simulink library "Lib_Solve_SSNRSolverBroydUpdate_TMATS"  (R2021b)
settings: Solver=ode45  StartTime=0.0  StopTime=10.0  RelTol=1e-3  EnableMultiTasking=on
libraries: Lib_NM_JacobianCalc_TMATS x1
Description:
  | Thomas Modules
settings Model: Creator=jwchapm2  LastModifiedBy=jwchapm2
settings SolverCC: AlgebraicLoopSolver=TrustRegion
settings DataIOCC: LimitDataPoints=on  SaveFormat=Array  ReturnWorkspaceOutputs=off
settings OptimizationCC: ExpressionDepthLimit=2147483647  LifeSpan=inf
settings DebuggingCC: UnderspecifiedInitializationDetection=Classic  MergeDetectMultiDrivingBlocksExec=none  SolverPrmCheckMsg=warning  StateNameClashWarn=warning  SFUnexpectedBacktrackingDiag=warning  SFNoUnconditionalDefaultTransitionDiag=warning  SFExecutionAtInitializationDiag=none  ArithmeticOperatorsInVariantConditions=warning
settings HardwareCC: ProdBitPerPointer=32  ProdBitPerSizeT=32  ProdBitPerPtrDiffT=32  ProdLargestAtomicFloat=None  ProdIntDivRoundTo=Undefined  ProdEndianess=Unspecified  ProdWordSize=32  ProdHWDeviceType=32-bit Generic
settings ModelReferenceCC: PropagateSignalLabelsOutOfModel=off
settings SFSimCC: SimUseLocalCustomCode=off  CustomCodeUndefinedFunction=UseInterfaceOnly
settings RTWCC: RTWUseLocalCustomCode=off
settings CodeAppCC: StateflowObjectComments=on
settings GRTTargetCC: TargetLangStandard=C89/C90 (ANSI)
settings ConfigComp: CovMetricSettings=dw  CovSaveCumulativeToWorkspaceVar=on  CovSaveSingleToWorkspaceVar=on  CovExternalEMLEnable=off

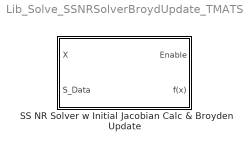
== system Lib_Solve_SSNRSolverBroydUpdate_TMATS ==
  SS NR Solver w Initial Jacobian Calc & Broyden Update : Subsystem  mask(T-MATS: SS NR Solver w Initial Jacobian Calc and Broyden Update Library Block){SJac_Per_M=[0.01 0.01 0.01;-0.01 -0.01,-0.01], SNR_IC_M=[1; 2; 3], SNR_DX_M=100, SNR_Mx_M=1000000, SNR_Mn_M=-1000000, Cond_Limits_M=0.0001}
      mask prompts: SJac_Per_M "SJac_Per_M - Jacobian Perturbation size (frac)(nxm)"; SNR_IC_M "SNR_IC_M - Newton Raphson Initial Conditions (mx1)"; SNR_DX_M "SNR_DX_M - Newton Raphson step size dampener. Percentage of calculated dx to use for each step (%) (1x1)"; SNR_Mx_M "SNR_Mx_M - Newton Raphson max limit (1x1 or mx1)"; SNR_Mn_M "SNR_Mn_M - Newton Raphson min limit (1x1 or mx1)"; Cond_Limits_M "Cond_Limits_M - Iteration Conditions Limits (mx1 or 1x1)"
      mask help:
      | The Steady State Newton Raphson Solver with Initial Jacobian Calculator and Broyden Update Method block will
      | supply the inputs to iteratively drive the outputs of a system to zero.
      |
      | This will be performed in three steps.
      | 1) Jabobian calculator sends Perturbations to the plant then calculates the initial plant
      | Jacboian based on the system response.
      | 2) The Newton Raphson Solver will use the inverse of the Jacobian to iteratively step the
      | system toward solution.
      | 3) The inverse of the Jacobian will be updated at each iteration via the Sherman-Morrison (Good) Broyden Update Method.
      | 3) Once the solution has satisfied the conditions the Newton Raphson Solver is shut off.
      |
      | Simulation run time length should be selected as to give the Newton Raphson Solver adequate time to develop a solution.
      mask init:
      | if isequal(size(SNR_Mx_M),size(SNR_IC_M))
      | elseif isequal(size(SNR_Mx_M),[1 1])
      | else
      |     disp('NR_Mx_Lim_M must be the same size as NR_IC_M or a constant')
      | end
      | 
      | if isequal(size(SNR_Mn_M),size(SNR_IC_M))
      | elseif isequal(size(SNR_Mn_M),[1 1])
      | else
      |     disp('NR_Mn_Lim_M must be the same size as NR_IC_M or a constant')
      | end
      mask Help: web(which('Solver_TMATS_SSNRwBU.html'),'-helpbrowser')

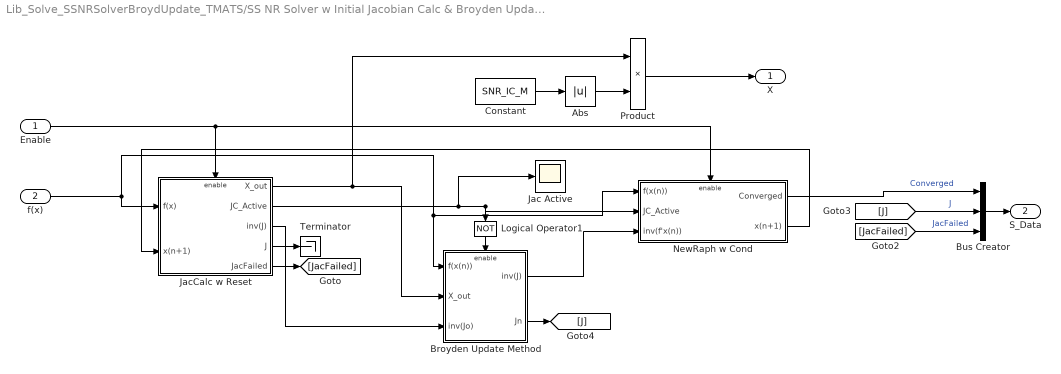
== system Lib_Solve_SSNRSolverBroydUpdate_TMATS/SS NR Solver w Initial Jacobian Calc & Broyden Update ==
  Enable : Inport  PortDimensions=1
  f(x) : Inport  Port=2  PortDimensions=length(SNR_IC_M)
  Abs : Abs
  Broyden Update Method : Subsystem
  Bus Creator : BusCreator  Inputs=3
  Constant : Constant  Value=SNR_IC_M
  Jac Active : Scope
  JacCalc w Reset : Subsystem  TreatAsAtomicUnit=on
  Logical Operator1 : Logic  Operator=NOT  AllPortsSameDT=off  OutDataTypeStr=boolean
  NewRaph w Cond : Subsystem  TreatAsAtomicUnit=on
  Product : Product  RndMeth=Zero
  Terminator : Terminator
  X : Outport  PortDimensions=length(SNR_IC_M)
  S_Data : Outport  Port=2  PortDimensions={1,[length(SNR_IC_M),length(SNR_IC_M)]}
  wires:
  Broyden Update Method/1("inv(J) ") -> NewRaph w Cond/3(inv(f'x(n)))
  Abs/1 -> Product/2
  Constant/1 -> Abs/1
  Product/1 -> X/1
  JacCalc w Reset/1(X_out) -> Broyden Update Method/2(X_out), Product/1
  Logical Operator1/1 -> Broyden Update Method/Enable
  Broyden Update Method/2(Jn) -> [J]
  JacCalc w Reset/2(JC_Active) -> NewRaph w Cond/2(JC_Active), Logical Operator1/1, Jac Active/1
  JacCalc w Reset/3(inv(J)) -> Broyden Update Method/3(inv(Jo))
  JacCalc w Reset/4(J) -> Terminator/1
  f(x)/1 -> NewRaph w Cond/1(f(x(n))), Broyden Update Method/1(f(x(n))), JacCalc w Reset/1(f(x))
  NewRaph w Cond/2(x(n+1)) -> JacCalc w Reset/2(x(n+1))
  NewRaph w Cond/1(Converged) -> Bus Creator/1  "Converged"
  Enable/1 -> NewRaph w Cond/Enable, JacCalc w Reset/Enable
  JacCalc w Reset/5(JacFailed) -> [JacFailed]
  Bus Creator/1 -> S_Data/1
  [J] -> Bus Creator/2  "J"
  [JacFailed] -> Bus Creator/3  "JacFailed"

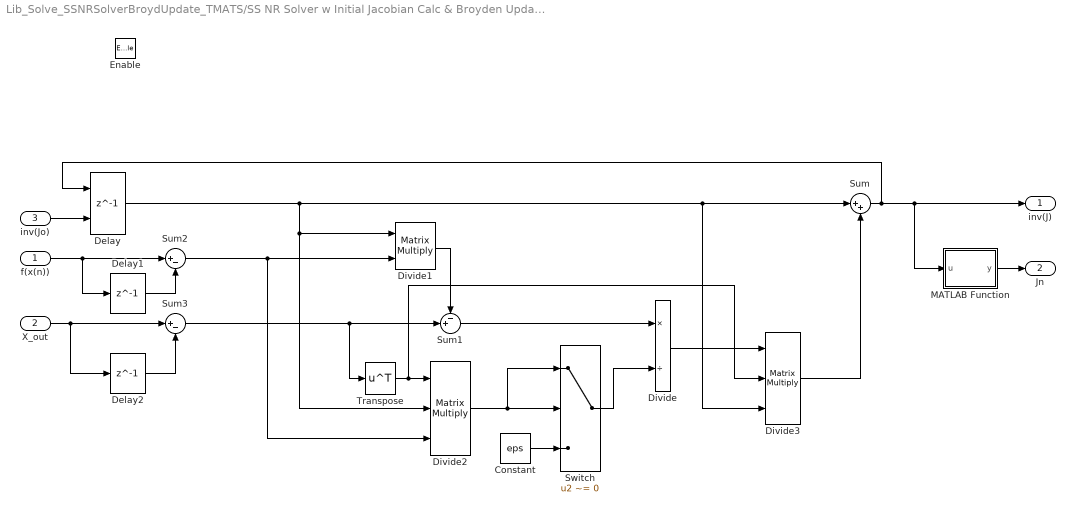
== system Lib_Solve_SSNRSolverBroydUpdate_TMATS/SS NR Solver w Initial Jacobian Calc & Broyden Update/Broyden Update Method ==
  f(x(n)) : Inport  PortDimensions=length(SNR_IC_M)
  X_out : Inport  Port=2  PortDimensions=length(SNR_IC_M)
  inv(Jo) : Inport  Port=3  PortDimensions=[length(SNR_IC_M),length(SNR_IC_M)]
  Enable : EnablePort
  Constant : Constant  Value=eps
  Delay : Delay  DelayLength=1  InitialConditionSource=Input port
      settings: InputPortMap=u0,p4
  Delay1 : Delay  DelayLength=1  InitialCondition=0
  Delay2 : Delay  DelayLength=1  InitialCondition=SNR_IC_M./abs(SNR_IC_M)
  Divide : Product  Inputs=*/
  Divide1 : Product  Inputs=**  Multiplication=Matrix(*)
  Divide2 : Product  Inputs=***  Multiplication=Matrix(*)
  Divide3 : Product  Inputs=***  Multiplication=Matrix(*)
  MATLAB Function : MATLAB Function  TreatAsAtomicUnit=on
  Sum : Sum  Inputs=|++
  Sum1 : Sum  Inputs=-+|
  Sum2 : Sum  Inputs=|+-
  Sum3 : Sum  Inputs=|+-
  Switch : Switch  Criteria=u2 ~= 0
  Transpose : Math  Operator=transpose  SaturateOnIntegerOverflow=on
  "inv(J) " : Outport  PortDimensions=[length(SNR_IC_M),length(SNR_IC_M)]
  Jn : Outport  Port=2  PortDimensions=[length(SNR_IC_M),length(SNR_IC_M)]
  wires:
  Delay2/1 -> Sum3/2
  inv(Jo)/1 -> Delay/2
  Delay/1 -> Divide3/3, Sum/1, Divide2/2, Divide1/1
  Delay1/1 -> Sum2/2
  f(x(n))/1 -> Sum2/1, Delay1/1
  Divide2/1 -> Switch/2, Switch/1
  Switch/1 -> Divide/2
  Sum3/1 -> Transpose/1, Sum1/2
  Constant/1 -> Switch/3
  Divide3/1 -> Sum/2
  Transpose/1 -> Divide3/2, Divide2/1
  X_out/1 -> Sum3/1, Delay2/1
  Sum2/1 -> Divide2/3, Divide1/2
  Divide/1 -> Divide3/1
  Sum1/1 -> Divide/1
  Divide1/1 -> Sum1/1
  Sum/1 -> Delay/1, "inv(J) "/1, MATLAB Function/1(u)
  MATLAB Function/1(y) -> Jn/1

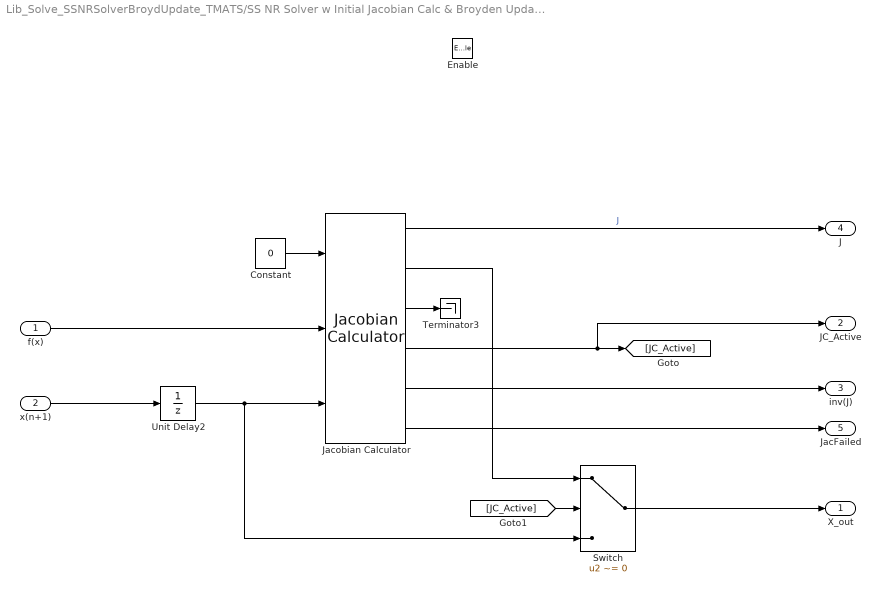
== system Lib_Solve_SSNRSolverBroydUpdate_TMATS/SS NR Solver w Initial Jacobian Calc & Broyden Update/JacCalc w Reset ==
  f(x) : Inport  PortDimensions=length(SNR_IC_M)
  x(n+1) : Inport  Port=2  PortDimensions=length(SNR_IC_M)
  Enable : EnablePort
  Constant : Constant  Value=0
  Jacobian Calculator : Lib_NM_JacobianCalc_TMATS/Jacobian Calculator  N_Per_M=SJac_Per_M
  Switch : Switch  Criteria=u2 ~= 0  Threshold=1
  Terminator3 : Terminator
  Unit Delay2 : UnitDelay  InitialCondition=SNR_IC_M./abs(SNR_IC_M)  SampleTime=-1  HasFrameUpgradeWarning=on
  X_out : Outport  PortDimensions=length(SNR_IC_M)
  JC_Active : Outport  Port=2  PortDimensions=1
  inv(J) : Outport  Port=3  PortDimensions=[length(SNR_IC_M),length(SNR_IC_M)]
  J : Outport  Port=4  PortDimensions=[length(SNR_IC_M),length(SNR_IC_M)]
  JacFailed : Outport  Port=5  PortDimensions=1
  wires:
  Constant/1 -> Jacobian Calculator/1
  Jacobian Calculator/3 -> Terminator3/1
  Jacobian Calculator/2 -> Switch/1
  Jacobian Calculator/4 -> [JC_Active], JC_Active/1
  Unit Delay2/1 -> Switch/3, Jacobian Calculator/3
  Jacobian Calculator/5 -> inv(J)/1
  Jacobian Calculator/1 -> J/1  "J"
  Switch/1 -> X_out/1
  x(n+1)/1 -> Unit Delay2/1
  [JC_Active] -> Switch/2
  f(x)/1 -> Jacobian Calculator/2
  Jacobian Calculator/6 -> JacFailed/1

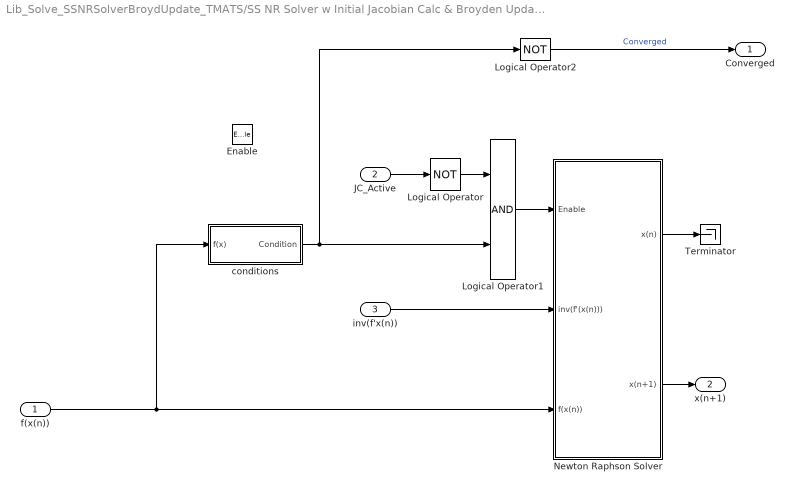
== system Lib_Solve_SSNRSolverBroydUpdate_TMATS/SS NR Solver w Initial Jacobian Calc & Broyden Update/NewRaph w Cond ==
  f(x(n)) : Inport  PortDimensions=length(SNR_IC_M)
  JC_Active : Inport  Port=2  PortDimensions=1
  inv(f'x(n)) : Inport  Port=3  PortDimensions=[length(SNR_IC_M),length(SNR_IC_M)]
  Enable : EnablePort
  Logical Operator : Logic  Operator=NOT  AllPortsSameDT=off  OutDataTypeStr=boolean
  Logical Operator1 : Logic  AllPortsSameDT=off  OutDataTypeStr=boolean
  Logical Operator2 : Logic  Operator=NOT  AllPortsSameDT=off  OutDataTypeStr=boolean
  Newton Raphson Solver : Subsystem  TreatAsAtomicUnit=on  mask(T-MATS: Newton Raphson Solver Library Block){NR_IC_M=SNR_IC_M./abs(SNR_IC_M), NR_dx_Damp_M=SNR_DX_M, NR_Mx_Lim_M=SNR_Mx_M./abs(SNR_IC_M), NR_Mn_Lim_M=SNR_Mn_M./abs(SNR_IC_M), BlkNm_M=double(gcb)}
      mask prompts: NR_IC_M "NR_IC_M - Initial Conditions of Newton Raphson (mx1)"; NR_dx_Damp_M "NR_dx_Damp_M - Newton Raphson step size dampener. Percentage of calculated dx to use for each step (%) (1x1)"; NR_Mx_Lim_M "NR_Mx_Lim_M - Max limit (1x1 or mx1)"; NR_Mn_Lim_M "NR_Mn_Lim_M - Min Limit (1x1 or mx1)"; BlkNm_M "BlkNm_M - Block Name"
      mask help:
      | Newton Raphson Solver:
      |
      | x(n+1) = x(n) - inverse(f'(x(n)))*f(x(n))
      |
      | Note:
      | inverse(f'(x(n))) is an m x m matrix and f(x(n)) is an m x 1 matrix
      | where m is the length of the initial conditions matrix and number of system independents.
      mask init:
      | if isequal(size(NR_Mx_Lim_M),size(NR_IC_M))
      | elseif isequal(size(NR_Mx_Lim_M),size(1))
      | else
      |     warning('NR_Mx_Lim_M must be the same size as NR_IC_M or a constant')
      | end
      | 
      | if isequal(size(NR_Mn_Lim_M),size(NR_IC_M))
      | elseif isequal(size(NR_Mn_Lim_M),size(1))
      | else
      |     warning('NR_Mn_Lim_M must be the same size as NR_IC_M or a constant')
      | end
      mask Help: web(which('NumMthd_TMATS_NRS.html'),'-helpbrowser')
  Terminator : Terminator
  conditions : Subsystem
  Converged : Outport  PortDimensions={1,[length(SNR_IC_M),length(SNR_IC_M)]}
  x(n+1) : Outport  Port=2  PortDimensions=length(SNR_IC_M)
  wires:
  Newton Raphson Solver/2(x(n+1)) -> x(n+1)/1
  JC_Active/1 -> Logical Operator/1
  Logical Operator/1 -> Logical Operator1/1
  Logical Operator1/1 -> Newton Raphson Solver/1(Enable)
  conditions/1(Condition) -> Logical Operator1/2, Logical Operator2/1
  Logical Operator2/1 -> Converged/1  "Converged"
  inv(f'x(n))/1 -> Newton Raphson Solver/2(inv(f'(x(n))))
  Newton Raphson Solver/1(x(n)) -> Terminator/1
  f(x(n))/1 -> conditions/1(f(x)), Newton Raphson Solver/3(f(x(n)))

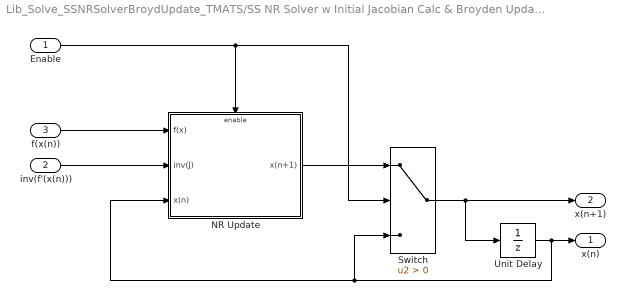
== system Lib_Solve_SSNRSolverBroydUpdate_TMATS/SS NR Solver w Initial Jacobian Calc & Broyden Update/NewRaph w Cond/Newton Raphson Solver ==
  Enable : Inport  PortDimensions=1
  inv(f'(x(n))) : Inport  Port=2  PortDimensions=[length(NR_IC_M),length(NR_IC_M)]
  f(x(n)) : Inport  Port=3  PortDimensions=length(NR_IC_M)
  NR Update : Subsystem
  Switch : Switch  Criteria=u2 > Threshold
  Unit Delay : UnitDelay  InitialCondition=NR_IC_M  SampleTime=-1  HasFrameUpgradeWarning=on
  x(n) : Outport  PortDimensions=length(NR_IC_M)
  x(n+1) : Outport  Port=2  PortDimensions=length(NR_IC_M)
  wires:
  Unit Delay/1 -> x(n)/1, Switch/3, NR Update/3(x(n))
  Enable/1 -> Switch/2, NR Update/Enable
  Switch/1 -> Unit Delay/1, x(n+1)/1
  f(x(n))/1 -> NR Update/1(f(x))
  inv(f'(x(n)))/1 -> NR Update/2(inv(J))
  NR Update/1(x(n+1)) -> Switch/1

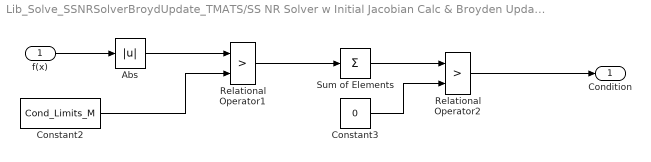
== system Lib_Solve_SSNRSolverBroydUpdate_TMATS/SS NR Solver w Initial Jacobian Calc & Broyden Update/NewRaph w Cond/conditions ==
  f(x) : Inport
  Abs : Abs
  Constant2 : Constant  Value=Cond_Limits_M
  Constant3 : Constant  Value=0
  Relational Operator1 : RelationalOperator  Operator=>  OutDataTypeStr=boolean  RndMeth=Nearest
  Relational Operator2 : RelationalOperator  Operator=>  OutDataTypeStr=boolean  RndMeth=Nearest
  Sum of Elements : Sum  Inputs=+
  Condition : Outport
  wires:
  Constant2/1 -> Relational Operator1/2
  Relational Operator1/1 -> Sum of Elements/1
  Constant3/1 -> Relational Operator2/2
  Abs/1 -> Relational Operator1/1
  Sum of Elements/1 -> Relational Operator2/1
  f(x)/1 -> Abs/1
  Relational Operator2/1 -> Condition/1

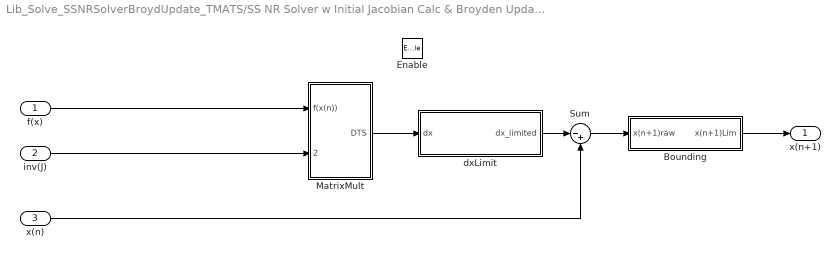
== system Lib_Solve_SSNRSolverBroydUpdate_TMATS/SS NR Solver w Initial Jacobian Calc & Broyden Update/NewRaph w Cond/Newton Raphson Solver/NR Update ==
  f(x) : Inport
  inv(J) : Inport  Port=2
  x(n) : Inport  Port=3
  Enable : EnablePort
  Bounding : Subsystem
  MatrixMult : Subsystem
  Sum : Sum  Inputs=|-+
  dxLimit : Subsystem
  x(n+1) : Outport
  wires:
  f(x)/1 -> MatrixMult/1(f(x(n)))
  Sum/1 -> Bounding/1(x(n+1)raw)
  MatrixMult/1(DTS) -> dxLimit/1(dx)
  dxLimit/1(dx_limited) -> Sum/1
  inv(J)/1 -> MatrixMult/2(inv(f'(x(n))))
  Bounding/1(x(n+1)Lim) -> x(n+1)/1
  x(n)/1 -> Sum/2

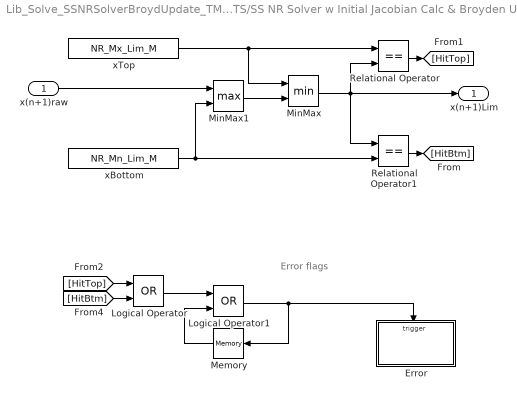
== system Lib_Solve_SSNRSolverBroydUpdate_TMATS/SS NR Solver w Initial Jacobian Calc & Broyden Update/NewRaph w Cond/Newton Raphson Solver/NR Update/Bounding ==
  note: Error flags
  x(n+1)raw : Inport
  Error : Subsystem
  Logical Operator : Logic  Operator=OR  AllPortsSameDT=off  OutDataTypeStr=boolean
  Logical Operator1 : Logic  Operator=OR  AllPortsSameDT=off  OutDataTypeStr=boolean
  Memory : Memory  InheritSampleTime=on
  MinMax : MinMax  Inputs=2
  MinMax1 : MinMax  Function=max  Inputs=2
  Relational Operator : RelationalOperator  Operator===  OutDataTypeStr=boolean  RndMeth=Nearest
  Relational Operator1 : RelationalOperator  Operator===  OutDataTypeStr=boolean  RndMeth=Nearest
  xBottom : Constant  Value=NR_Mn_Lim_M
  xTop : Constant  Value=NR_Mx_Lim_M
  x(n+1)Lim : Outport
  wires:
  xBottom/1 -> MinMax1/2, Relational Operator1/2
  x(n+1)raw/1 -> MinMax1/1
  xTop/1 -> Relational Operator/1, MinMax/1
  MinMax1/1 -> MinMax/2
  MinMax/1 -> Relational Operator1/1, Relational Operator/2, x(n+1)Lim/1
  Relational Operator1/1 -> [HitBtm]
  Relational Operator/1 -> [HitTop]
  [HitTop] -> Logical Operator/1
  Logical Operator/1 -> Logical Operator1/1
  [HitBtm] -> Logical Operator/2
  Memory/1 -> Logical Operator1/2
  Logical Operator1/1 -> Error/Trigger, Memory/1

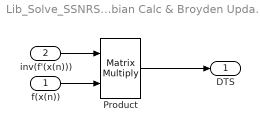
== system Lib_Solve_SSNRSolverBroydUpdate_TMATS/SS NR Solver w Initial Jacobian Calc & Broyden Update/NewRaph w Cond/Newton Raphson Solver/NR Update/MatrixMult ==
  f(x(n)) : Inport
  inv(f'(x(n))) : Inport  Port=2
  Product : Product  Multiplication=Matrix(*)  RndMeth=Zero
  DTS : Outport
  wires:
  Product/1 -> DTS/1
  f(x(n))/1 -> Product/2
  inv(f'(x(n)))/1 -> Product/1

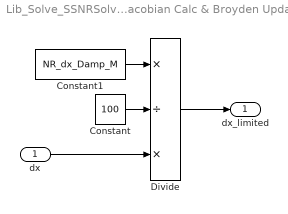
== system Lib_Solve_SSNRSolverBroydUpdate_TMATS/SS NR Solver w Initial Jacobian Calc & Broyden Update/NewRaph w Cond/Newton Raphson Solver/NR Update/dxLimit ==
  dx : Inport
  Constant : Constant  Value=100
  Constant1 : Constant  Value=NR_dx_Damp_M
  Divide : Product  Inputs=*/*
  dx_limited : Outport
  wires:
  Divide/1 -> dx_limited/1
  Constant1/1 -> Divide/1
  Constant/1 -> Divide/2
  dx/1 -> Divide/3

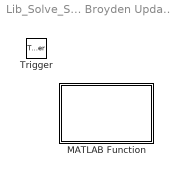
== system Lib_Solve_SSNRSolverBroydUpdate_TMATS/SS NR Solver w Initial Jacobian Calc & Broyden Update/NewRaph w Cond/Newton Raphson Solver/NR Update/Bounding/Error ==
  Trigger : TriggerPort  VariantControl=(inherit)
  MATLAB Function : MATLAB Function  TreatAsAtomicUnit=on

== matlab function Lib_Solve_SSNRSolverBroydUpdate_TMATS/SS NR Solver w Initial Jacobian Calc & Broyden Update/NewRaph w Cond/Newton Raphson Solver/NR Update/Bounding/Error/MATLAB Function ==
  data: BlkNm_M parameter
function fcn(BlkNm_M)
%# Limit Newton Raphson outputs and produce a warning if it occurs
BName = BlkNm_M;
disp(['Warning in ' BName ': Solver limit has been hit, check for system convergence']);

== matlab function Lib_Solve_SSNRSolverBroydUpdate_TMATS/SS NR Solver w Initial Jacobian Calc & Broyden Update/Broyden Update Method/MATLAB Function ==
  data: u input; y output
function y = Inverse(u)

y = inv(u);
